simulink model "GainCompensatedUnityFeedbackResponse"  (R2020b)
settings: Solver=FixedStepAuto  StartTime=0.0  StopTime=10  FixedStep=0.001  RelTol=1e-3
undefined symbols (not defined in the file): b, I, l, M, m
settings Model: Creator=jdavis6874  LastModifiedBy=jdavis6874
settings SFSimCC: CustomCodeUndefinedFunction=UseInterfaceOnly

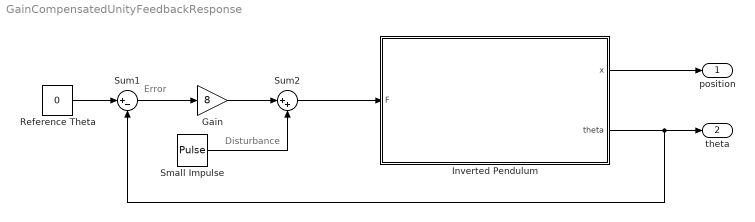
== system GainCompensatedUnityFeedbackResponse ==
  note: Disturbance
  note: Error
  Gain : Gain  Gain=8
  Inverted Pendulum : Subsystem
  Reference Theta : Constant  Value=0
  Small Impulse : DiscretePulseGenerator  PulseType=Time based  Amplitude=1000  Period=100  PulseWidth=0.001
  Sum1 : Sum  Inputs=|+-
  Sum2 : Sum  Inputs=|++
  position : Outport  VectorParamsAs1DForOutWhenUnconnected=off
  theta : Outport  Port=2  VectorParamsAs1DForOutWhenUnconnected=off
  wires:
  Inverted Pendulum/1(x) -> position/1
  Inverted Pendulum/2(theta) -> Sum1/2, theta/1
  Reference Theta/1 -> Sum1/1
  Sum2/1 -> Inverted Pendulum/1(F)
  Small Impulse/1 -> Sum2/2
  Sum1/1 -> Gain/1
  Gain/1 -> Sum2/1

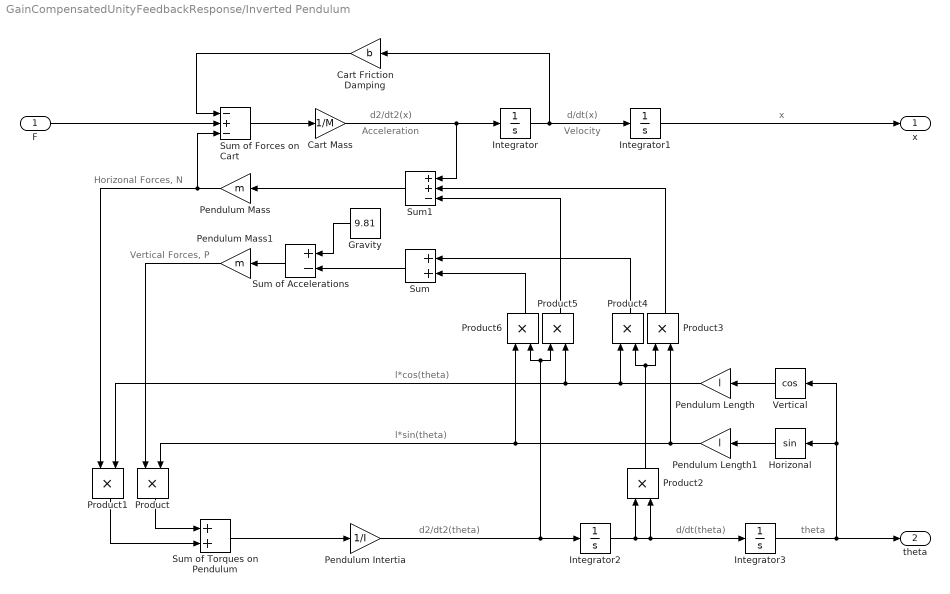
== system GainCompensatedUnityFeedbackResponse/Inverted Pendulum ==
  note: d2/dt2(x)
  note: d/dt(x)
  note: Horizonal Forces, N
  note: d2/dt2(theta)
  note: Vertical Forces, P
  note: Acceleration
  note: x
  note: l*cos(theta)
  note: theta
  note: Velocity
  note: d/dt(theta)
  note: l*sin(theta)
  F : Inport
  Cart Friction Damping : Gain  Gain=b
  Cart Mass : Gain  Gain=1/M
  Gravity : Constant  Value=9.81
  Horizonal : Trigonometry
  Integrator{,1..3} (4 alike) : Integrator
  Pendulum Intertia : Gain  Gain=1/I
  Pendulum Length : Gain  Gain=l
  Pendulum Length1 : Gain  Gain=l
  Pendulum Mass : Gain  Gain=m
  Pendulum Mass1 : Gain  Gain=m
  Product{,1..6} (7 alike) : Product
  Sum : Sum
  Sum of Accelerations : Sum  Inputs=+-
  Sum of Forces on Cart : Sum  Inputs=-+-
  Sum of Torques on Pendulum : Sum
  Sum1 : Sum  Inputs=++-
  Vertical : Trigonometry  Operator=cos
  x : Outport  VectorParamsAs1DForOutWhenUnconnected=off
  theta : Outport  Port=2  VectorParamsAs1DForOutWhenUnconnected=off
  wires:
  Sum of Torques on Pendulum/1 -> Pendulum Intertia/1
  Integrator2/1 -> Product2/1, Product2/2, Integrator3/1
  Pendulum Intertia/1 -> Product6/2, Product5/1, Integrator2/1
  Cart Friction Damping/1 -> Sum of Forces on Cart/1
  Product4/1 -> Sum/1
  Product/1 -> Sum of Torques on Pendulum/1
  Pendulum Mass1/1 -> Product/1
  Product1/1 -> Sum of Torques on Pendulum/2
  Product5/1 -> Sum1/3
  Cart Mass/1 -> Sum1/1, Integrator/1
  Integrator/1 -> Cart Friction Damping/1, Integrator1/1
  Product3/1 -> Sum1/2
  Integrator3/1 -> theta/1, Vertical/1, Horizonal/1
  Product2/1 -> Product3/1, Product4/2
  Vertical/1 -> Pendulum Length/1
  Pendulum Length1/1 -> Product3/2, Product6/1, Product/2
  Product6/1 -> Sum/2
  Horizonal/1 -> Pendulum Length1/1
  Pendulum Mass/1 -> Sum of Forces on Cart/3, Product1/1
  Pendulum Length/1 -> Product4/1, Product5/2, Product1/2
  F/1 -> Sum of Forces on Cart/2
  Sum of Accelerations/1 -> Pendulum Mass1/1
  Sum1/1 -> Pendulum Mass/1
  Sum/1 -> Sum of Accelerations/2
  Sum of Forces on Cart/1 -> Cart Mass/1
  Integrator1/1 -> x/1
  Gravity/1 -> Sum of Accelerations/1
